simulink model "Tarea_1_P2"  (R2024b)
settings: Solver=VariableStepAuto  StartTime=0.0  StopTime=10.0  RelTol=1e-3
settings Model: Creator=Usuario  LastModifiedBy=Lenovo

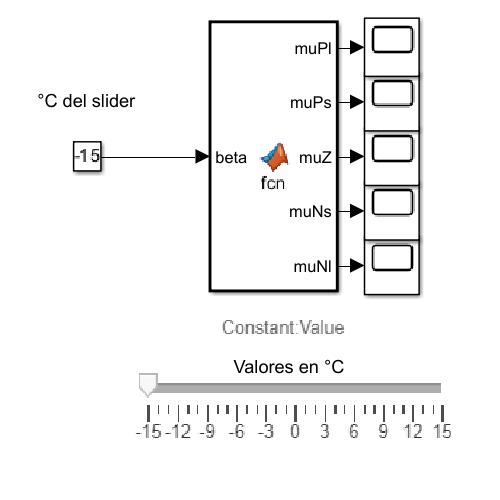
[thumbnail: Simulink's stored preview of the top-level diagram]
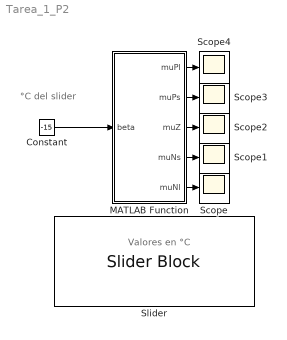
== system Tarea_1_P2 ==
  note: °C del slider
  note: Valores en °C
  Constant : Constant  Value=-15
  MATLAB Function : MATLAB Function  TreatAsAtomicUnit=on
  Scope{,1..4} (5 alike) : Scope
  Slider : SliderBlock  ScaleMin=-15  ScaleMax=15
  wires:
  Constant/1 -> MATLAB Function/1(beta)
  MATLAB Function/3(muZ) -> Scope2/1
  MATLAB Function/5(muNl) -> Scope/1
  MATLAB Function/4(muNs) -> Scope1/1
  MATLAB Function/2(muPs) -> Scope3/1
  MATLAB Function/1(muPl) -> Scope4/1

== matlab function Tarea_1_P2/MATLAB Function ==
  data: muPl output; muPs output; muZ output; muNs output; muNl output; beta input
function [muPl, muPs, muZ, muNs, muNl] = fcn(beta)

% Para μ Positivo Large
if beta <= 7.5
    muPl = 0;
elseif beta > 7.5 && beta <= 15
    muPl = (beta - 7.5)/7.5;
else
    muPl = 1;
end

% Para μ Positivo Small
if beta <= 0
    muPs = 0;
elseif beta > 0 && beta <= 7.5
    muPs = beta/7.5;
elseif beta > 7.5 && beta <= 15
    muPs = (15 - beta)/7.5;
else
    muPs = 0;
end
%  Para μ Zero
if beta <= -7.5
    muZ = 0;
elseif beta > -7.5 && beta <= 0
    muZ = (beta + 7.5)/7.5;
elseif beta > 0 && beta <= 7.5
    muZ = (7.5 - beta)/7.5;
else
    muZ = 0;
end
% Para μ Negativo Small
if beta <= -15
    muNs = 0;
elseif beta > -15 && beta <= -7.5
    muNs = (beta + 15)/7.5;
elseif beta > -7.5 && beta <= 0
    muNs = -beta/7.5;
else
    muNs = 0;
end
% Para μ Negativo Large
if beta <= -15
    muNl = 1;
elseif beta > -15 && beta <= -7.5
    muNl = (-7.5 - beta)/7.5;
else
    muNl = 0;
end

end
